simulink model "V2X_Core_SRI_coding_rate_symbol"  (R2023b)
settings: Solver=ode23tb  StartTime=0.0  StopTime=50  MaxStep=1e-2  RelTol=1e-3  AbsTol=1e-3
StopFcn:
  | run('saving.m')
values from neighbouring files (symbols this model uses):
  b = 1.6    [a2024_v2x_matlab_6veh.m]
  m = 2000    [a2024_v2x_matlab_6veh.m]
  mEgo = 1500    [a2024_v2x_matlab_6veh.m]
  Mode = 1    [a2024_v2x_matlab_6veh.m]    (also in v2x_matlab.m; v2x_matlabV2.m; v2x_matlab_6veh.m; v2x_matlab_R.m)
  RefSpeed = 90/3.6    (= 25)    [v2x_matlabV2.m]    (also in v2x_matlab_R.m)
  RelDistThreshold = 300    [v2x_matlabV2.m]    (also in v2x_matlab_R.m)
  s = RandStream("dsfmt19937","Seed",15)    [v2x_matlab.m]
  sampleTime = 0.1    [a2024_v2x_matlab_6veh.m]    (also in v2x_matlab.m; v2x_matlabV2.m; v2x_matlab_6veh.m; v2x_matlab_R.m)
  waypoints = [egoWP(:,2) egoWP(:,1), zeroforwp]    [a2024_v2x_matlab_6veh.m]    (also in misc.m = data.data.ActorSpecifications(1,1).Waypoints(:,[1,2]); v2x_matlab.m = data.data.ActorSpecifications(1,1).Waypoints(:,[1,2]); v2x_matlabV2.m = [5 -1.6 0; v2x_matlab_R.m = [5 -1.6 0)
  ZeroActors = struct(     'ActorID',0,     'Position', [1000 1000 1000],      'Velocity', [0 0 0],      'Roll', 0,      'Pitch', 0,      'Yaw', 0,      'AngularVelocity', [0 0 0])    [v2x_matlabV2.m]    (also in v2x_matlab_R.m)
undefined symbols (not defined in the file or in its folder): Battery, Brakes, Control, DiscIntNeverNeededParam, doppler, Drivetrain, ElectricMotor, Env, FB_flag, Init, SNR_value_list, Vehicle, Wheels
libraries: simulink x45, commofdm x29, commdigbbndam3 x15, commchan3 x14, simulink_extras x13, commcnvcod2 x12, commdigbbndpm3 x11, commblkintrlv2 x10, dspmathops x6, sharedtransform x6, autolibutils x6, autolibsharedcoupling x4
(part 5 of 8)

== system V2X_Core_SRI_coding_rate_symbol/DSRC/Subsystem/2//3 64 QAM ==
  Bits : Inport
  Pilot : Inport  Port=2
  Constant2 : Constant  Value=[zeros(24,1)']  SampleTime=-1
  Convolutional Encoder1 : commcnvcod2/Convolutional Encoder  trellis=poly2trellis(7, [171 133])  opMode=Truncated (reset every frame)  DelayedResetAction=on  hasIniStPort=off  hasFinStPort=off  usePuncVector=on  punctureVector=[1; 1; 0; 1]  reset=Unused parameter value
      settings: LibrarySourceBlock=|
      | commhdlcnvcod/Convolutional
      | Encoder
  Gain : Gain  Gain=1/sqrt(5)
  OFDM Modulator1 : commofdm/OFDM Modulator  StatePerturbationForJacobian=1.0e-05  FFTLength=64  NumGuardBandCarriers=[6; 5]  InsertDCNull=on  PilotInputPort=on  PilotCarrierIndices=[12; 26; 40; 54]  CyclicPrefixLength=16  Windowing=off  WindowLength=1  OversamplingFactor=1  NumSymbols=2  NumTransmitAntennas=1  SimulateUsing=Interpreted execution
  Random Interleaver : commblkintrlv2/Random Interleaver  StatePerturbationForJacobian=1.0e-05  N=432  seed=12345
  Rectangular QAM Modulator Baseband2 : commdigbbndam3/Rectangular QAM Modulator Baseband  M=2^6  InType=Bit  Enc=Gray  Mapping=[0:15]  PowType=Average Power  MinDist=2  AvgPow=1  PeakPow=42  Ph=0  outDtype=double  outWordLen=16  outUDDataType=sfix(16)  outFracLenMode=Best precision  outFracLen=15  outDataTypeStr=double  outLastDataTypeStr=double
      settings: LibrarySourceBlock=|
      | commhdldigbbndam/Rectangular QAM
      | Modulator
      | Baseband
  Reshape : Reshape  OutputDimensionality=Customize  OutputDimensions=[48,2]
  Vector Concatenate : Concatenate
  Modulated : Outport
  wires:
  Convolutional Encoder1/1 -> Random Interleaver/1
  OFDM Modulator1/1 -> Modulated/1  "OFDM modulated"
  Pilot/1 -> OFDM Modulator1/2
  Vector Concatenate/1 -> Reshape/1  "After QAM Mod"
  Constant2/1 -> Vector Concatenate/2
  Random Interleaver/1 -> Rectangular QAM Modulator Baseband2/1
  Reshape/1 -> OFDM Modulator1/1
  Bits/1 -> Convolutional Encoder1/1
  Rectangular QAM Modulator Baseband2/1 -> Gain/1
  Gain/1 -> Vector Concatenate/1

== system V2X_Core_SRI_coding_rate_symbol/DSRC/Subsystem/2//3 64 QAM1 ==
  Bits : Inport
  Pilot : Inport  Port=2
  Constant2 : Constant  Value=[zeros(24,1)']  SampleTime=-1
  Convolutional Encoder1 : commcnvcod2/Convolutional Encoder  trellis=poly2trellis(7, [171 133])  opMode=Truncated (reset every frame)  DelayedResetAction=on  hasIniStPort=off  hasFinStPort=off  usePuncVector=on  punctureVector=[1; 1; 0; 1]  reset=Unused parameter value
      settings: LibrarySourceBlock=|
      | commhdlcnvcod/Convolutional
      | Encoder
  OFDM Modulator1 : commofdm/OFDM Modulator  StatePerturbationForJacobian=1.0e-05  FFTLength=64  NumGuardBandCarriers=[6; 5]  InsertDCNull=on  PilotInputPort=on  PilotCarrierIndices=[12; 26; 40; 54]  CyclicPrefixLength=16  Windowing=off  WindowLength=1  OversamplingFactor=1  NumSymbols=2  NumTransmitAntennas=1  SimulateUsing=Interpreted execution
  OFDM Modulator2 : commofdm/OFDM Modulator  Commented=on  StatePerturbationForJacobian=1.0e-05  FFTLength=1024  NumGuardBandCarriers=[0;0]  InsertDCNull=on  PilotInputPort=on  PilotCarrierIndices=[128; 256; 384; 640; 768; 896]  CyclicPrefixLength=256  Windowing=off  WindowLength=16  OversamplingFactor=3  NumSymbols=1  NumTransmitAntennas=1  SimulateUsing=Interpreted execution
  Rectangular QAM Modulator Baseband2 : commdigbbndam3/Rectangular QAM Modulator Baseband  M=2^6  InType=Bit  Enc=Gray  Mapping=[0:15]  PowType=Average Power  MinDist=2  AvgPow=42  PeakPow=1  Ph=0  outDtype=double  outWordLen=16  outUDDataType=sfix(16)  outFracLenMode=Best precision  outFracLen=15  outDataTypeStr=double  outLastDataTypeStr=double
      settings: LibrarySourceBlock=|
      | commhdldigbbndam/Rectangular QAM
      | Modulator
      | Baseband
  Reshape : Reshape  OutputDimensionality=Customize  OutputDimensions=[48,2]
  Vector Concatenate : Concatenate
  Modulated : Outport
  wires:
  Constant2/1 -> Vector Concatenate/2
  Vector Concatenate/1 -> Reshape/1  "After QAM Mod"
  Pilot/1 -> OFDM Modulator1/2
  Rectangular QAM Modulator Baseband2/1 -> Vector Concatenate/1
  OFDM Modulator1/1 -> Modulated/1  "OFDM modulated"
  Bits/1 -> Convolutional Encoder1/1
  Convolutional Encoder1/1 -> Rectangular QAM Modulator Baseband2/1
  Reshape/1 -> OFDM Modulator1/1

== system V2X_Core_SRI_coding_rate_symbol/DSRC/Subsystem/3//4 64 QAM ==
  Bits : Inport
  Pilot : Inport  Port=2
  Constant2 : Constant  Value=[zeros(32,1)']  SampleTime=-1
  Convolutional Encoder1 : commcnvcod2/Convolutional Encoder  trellis=poly2trellis(7, [171 133])  opMode=Truncated (reset every frame)  DelayedResetAction=on  hasIniStPort=off  hasFinStPort=off  usePuncVector=on  punctureVector=[1; 1; 0; 1; 1; 0]  reset=Unused parameter value
      settings: LibrarySourceBlock=|
      | commhdlcnvcod/Convolutional
      | Encoder
  OFDM Modulator1 : commofdm/OFDM Modulator  StatePerturbationForJacobian=1.0e-05  FFTLength=64  NumGuardBandCarriers=[6; 5]  InsertDCNull=on  PilotInputPort=on  PilotCarrierIndices=[12; 26; 40; 54]  CyclicPrefixLength=16  Windowing=off  WindowLength=1  OversamplingFactor=1  NumSymbols=2  NumTransmitAntennas=1  SimulateUsing=Interpreted execution
  Random Interleaver : commblkintrlv2/Random Interleaver  StatePerturbationForJacobian=1.0e-05  N=384  seed=12345
  Rectangular QAM Modulator Baseband2 : commdigbbndam3/Rectangular QAM Modulator Baseband  M=2^6  InType=Bit  Enc=Gray  Mapping=[0:15]  PowType=Average Power  MinDist=2  AvgPow=0.2  PeakPow=1  Ph=0  outDtype=double  outWordLen=16  outUDDataType=sfix(16)  outFracLenMode=Best precision  outFracLen=15  outDataTypeStr=double  outLastDataTypeStr=double
      settings: LibrarySourceBlock=|
      | commhdldigbbndam/Rectangular QAM
      | Modulator
      | Baseband
  Reshape : Reshape  OutputDimensionality=Customize  OutputDimensions=[48,2]
  Vector Concatenate : Concatenate
  Modulated : Outport
  wires:
  Constant2/1 -> Vector Concatenate/2
  Vector Concatenate/1 -> Reshape/1  "After QAM Mod"
  Pilot/1 -> OFDM Modulator1/2
  Rectangular QAM Modulator Baseband2/1 -> Vector Concatenate/1
  OFDM Modulator1/1 -> Modulated/1  "OFDM modulated"
  Bits/1 -> Convolutional Encoder1/1
  Convolutional Encoder1/1 -> Random Interleaver/1
  Random Interleaver/1 -> Rectangular QAM Modulator Baseband2/1
  Reshape/1 -> OFDM Modulator1/1

== system V2X_Core_SRI_coding_rate_symbol/DSRC/Subsystem/3//4 QPSK ==
  Bits : Inport
  Pilot : Inport  Port=2
  Constant : Constant  Commented=on  Value=zeros(0,1)
  Convolutional Encoder1 : commcnvcod2/Convolutional Encoder  trellis=poly2trellis(7, [171 133])  opMode=Truncated (reset every frame)  DelayedResetAction=on  hasIniStPort=off  hasFinStPort=off  usePuncVector=on  punctureVector=[1; 1; 0; 1; 1; 0]  reset=Unused parameter value
      settings: LibrarySourceBlock=|
      | commhdlcnvcod/Convolutional
      | Encoder
  Gain : Gain  Gain=1/sqrt(5)
  OFDM Modulator : commofdm/OFDM Modulator  StatePerturbationForJacobian=1.0e-05  FFTLength=64  NumGuardBandCarriers=[6; 5]  InsertDCNull=on  PilotInputPort=on  PilotCarrierIndices=[12; 26; 40; 54]  CyclicPrefixLength=16  Windowing=off  WindowLength=1  OversamplingFactor=1  NumSymbols=4  NumTransmitAntennas=1  SimulateUsing=Interpreted execution
  QPSK Modulator Baseband : commdigbbndpm3/QPSK Modulator Baseband  InType=Bit  Enc=Gray  Ph=pi/4  outDtype=double  outWordLen=16  outUDDataType=sfix(16)  outFracLenMode=Best precision  outFracLen=15  outDataTypeStr=double  outLastDataTypeStr=double
      settings: LibrarySourceBlock=|
      | commhdldigbbndpm/QPSK
      | Modulator
      | Baseband
  Random Interleaver : commblkintrlv2/Random Interleaver  StatePerturbationForJacobian=1.0e-05  N=384  seed=12345
  Reshape : Reshape  OutputDimensionality=Customize  OutputDimensions=[48,4]
  Vector Concatenate : Concatenate  Commented=on
  Modulated : Outport
  wires:
  OFDM Modulator/1 -> Modulated/1  "OFDM modulated"
  Pilot/1 -> OFDM Modulator/2
  Bits/1 -> Convolutional Encoder1/1
  Constant/1 -> Vector Concatenate/2
  Convolutional Encoder1/1 -> Random Interleaver/1
  Random Interleaver/1 -> QPSK Modulator Baseband/1
  QPSK Modulator Baseband/1 -> Gain/1
  Reshape/1 -> OFDM Modulator/1
  Gain/1 -> Reshape/1

== system V2X_Core_SRI_coding_rate_symbol/DSRC/Subsystem3/1//2 QPSK ==
  Output : Inport
  Bit to Integer Converter2 : simulink/Logic and Bit Operations/Bit to Integer Converter  nbits=16  bitOrder=MSB first  signedOutputValues=Signed  outDtype=int16  outDtypeSigned=int16
  Display : Display
  OFDM Demodulator1 : commofdm/OFDM Demodulator  StatePerturbationForJacobian=1.0e-05  FFTLength=64  NumGuardBandCarriers=[6; 5]  RemoveDCCarrier=on  PilotOutputPort=on  PilotCarrierIndices=[12; 26; 40; 54]  CyclicPrefixLength=16  OversamplingFactor=1  NumSymbols=6  NumReceiveAntennas=1  SimulateUsing=Interpreted execution
  QPSK Demodulator Baseband : commdigbbndpm3/QPSK Demodulator Baseband  OutType=Bit  DecType=Hard decision  VarSource=Dialog  Variance=1  Dec=Gray  Ph=pi/4  outDtype1=Inherit via internal rule  outDtype2=Inherit via internal rule  derotateFactorWordLen=16  derotateFactorDataTypeStr=Inherit: Same word length as input  derotateFactorLastDataTypeStr=Inherit: Same word length as input
      settings: LibrarySourceBlock=|
      | commhdldigbbndpm/QPSK
      | Demodulator
      | Baseband
  Random Deinterleaver : commblkintrlv2/Random Deinterleaver  StatePerturbationForJacobian=1.0e-05  N=576  seed=12345
  Reshape : Reshape
  Selector : Selector  InputPortWidth=288  IndexOptions=Index vector (dialog)  Indices=[1:288]  OutputSizes=1
  Viterbi Decoder : commcnvcod2/Viterbi Decoder  trellis=poly2trellis(7, [171 133])  isPunctured=off  punctureVector=[1; 1; 0; 1; 1; 0]  erasures=off  dectype=Hard decision  nsdecb=4  runSigValErrCheck=off  tbdepth=30  opmode=Truncated  reset=off  delayedResetAction=on  smWordLength=16  outDataType=Smallest unsigned integer
      settings: LibrarySourceBlock=commhdlcnvcod/Viterbi Decoder
  Modulated : Outport
  wires:
  OFDM Demodulator1/2 -> Display/1
  OFDM Demodulator1/1 -> Reshape/1  "Before QAM Demod"
  Output/1 -> OFDM Demodulator1/1
  QPSK Demodulator Baseband/1 -> Random Deinterleaver/1
  Selector/1 -> QPSK Demodulator Baseband/1
  Bit to Integer Converter2/1 -> Modulated/1
  Viterbi Decoder/1 -> Bit to Integer Converter2/1
  Random Deinterleaver/1 -> Viterbi Decoder/1
  Reshape/1 -> Selector/1

== system V2X_Core_SRI_coding_rate_symbol/DSRC/Subsystem3/1//2 QPSK1 ==
  Output : Inport
  Bit to Integer Converter2 : simulink/Logic and Bit Operations/Bit to Integer Converter  nbits=16  bitOrder=MSB first  signedOutputValues=Signed  outDtype=int16  outDtypeSigned=int16
  Display : Display
  OFDM Demodulator1 : commofdm/OFDM Demodulator  Commented=on  StatePerturbationForJacobian=1.0e-05  FFTLength=64  NumGuardBandCarriers=[0; 0]  RemoveDCCarrier=on  PilotOutputPort=on  PilotCarrierIndices=[12; 26; 40; 54]  CyclicPrefixLength=32  OversamplingFactor=3  NumSymbols=1  NumReceiveAntennas=1  SimulateUsing=Interpreted execution
  OFDM Demodulator2 : commofdm/OFDM Demodulator  StatePerturbationForJacobian=1.0e-05  FFTLength=64  NumGuardBandCarriers=[6; 5]  RemoveDCCarrier=on  PilotOutputPort=on  PilotCarrierIndices=[12; 26; 40; 54]  CyclicPrefixLength=16  OversamplingFactor=1  NumSymbols=6  NumReceiveAntennas=1  SimulateUsing=Interpreted execution
  QPSK Demodulator Baseband : commdigbbndpm3/QPSK Demodulator Baseband  OutType=Bit  DecType=Hard decision  VarSource=Dialog  Variance=1  Dec=Gray  Ph=pi/4  outDtype1=Inherit via internal rule  outDtype2=Inherit via internal rule  derotateFactorWordLen=16  derotateFactorDataTypeStr=Inherit: Same word length as input  derotateFactorLastDataTypeStr=Inherit: Same word length as input
      settings: LibrarySourceBlock=|
      | commhdldigbbndpm/QPSK
      | Demodulator
      | Baseband
  Random Deinterleaver : commblkintrlv2/Random Deinterleaver  StatePerturbationForJacobian=1.0e-05  N=576  seed=12345
  Reshape : Reshape
  Selector : Selector  InputPortWidth=288  IndexOptions=Index vector (dialog)  Indices=[1:288]  OutputSizes=1
  Viterbi Decoder : commcnvcod2/Viterbi Decoder  trellis=poly2trellis(7, [171 133])  isPunctured=off  punctureVector=[1; 1; 0; 1; 1; 0]  erasures=off  dectype=Hard decision  nsdecb=4  runSigValErrCheck=off  tbdepth=30  opmode=Truncated  reset=off  delayedResetAction=on  smWordLength=16  outDataType=Smallest unsigned integer
      settings: LibrarySourceBlock=commhdlcnvcod/Viterbi Decoder
  Modulated : Outport
  wires:
  Viterbi Decoder/1 -> Bit to Integer Converter2/1
  Bit to Integer Converter2/1 -> Modulated/1
  Selector/1 -> QPSK Demodulator Baseband/1
  QPSK Demodulator Baseband/1 -> Random Deinterleaver/1
  Output/1 -> OFDM Demodulator2/1
  OFDM Demodulator2/1 -> Reshape/1  "Before QAM Demod"
  OFDM Demodulator2/2 -> Display/1
  Reshape/1 -> Selector/1
  Random Deinterleaver/1 -> Viterbi Decoder/1

== system V2X_Core_SRI_coding_rate_symbol/DSRC/Subsystem3/2//3 64 QAM ==
  Output : Inport
  Bit to Integer Converter2 : simulink/Logic and Bit Operations/Bit to Integer Converter  nbits=16  bitOrder=MSB first  signedOutputValues=Signed  outDtype=int16  outDtypeSigned=int16
  Display : Display
  Display1 : Display
  MATLAB Function3 : MATLAB Function  Commented=on  TreatAsAtomicUnit=on
  OFDM Demodulator1 : commofdm/OFDM Demodulator  StatePerturbationForJacobian=1.0e-05  FFTLength=64  NumGuardBandCarriers=[6; 5]  RemoveDCCarrier=on  PilotOutputPort=on  PilotCarrierIndices=[12; 26; 40; 54]  CyclicPrefixLength=16  OversamplingFactor=1  NumSymbols=2  NumReceiveAntennas=1  SimulateUsing=Interpreted execution
  Random Deinterleaver : commblkintrlv2/Random Deinterleaver  StatePerturbationForJacobian=1.0e-05  N=432  seed=12345
  Rectangular QAM Demodulator Baseband2 : commdigbbndam3/Rectangular QAM Demodulator Baseband  M=2^6  OutType=Bit  DecType=Hard decision  VarSource=Dialog  Variance=1  Dec=Gray  Mapping=[0:15]  PowType=Average Power  MinDist=2  AvgPow=0.2  PeakPow=1  Ph=0  outDtype1=int16  outDtype2=int16  derotateFactorWordLen=16  derotateFactorDataTypeStr=Inherit: Same word length as input  derotateFactorLastDataTypeStr=Inherit: Same word length as input  denormFactorWordLen=16  denormFactorDataTypeStr=Inherit: Same word length as input  denormFactorLastDataTypeStr=Inherit: Same word length as input  prodOutWordLen=32  prodOutOverflowMode=Wrap  prodOutRoundingMode=Floor  prodOutOvFlMode=off  prodOutOvFlModeLastStrValue=off  sumWordLen=32
      settings: LibrarySourceBlock=|
      | commhdldigbbndam/Rectangular QAM
      | Demodulator
      | Baseband
  Reshape : Reshape
  Selector : Selector  InputPortWidth=96  IndexOptions=Index vector (dialog)  Indices=[1:72]  OutputSizes=1
  Viterbi Decoder : commcnvcod2/Viterbi Decoder  trellis=poly2trellis(7, [171 133])  isPunctured=on  punctureVector=[1; 1; 0; 1]  erasures=off  dectype=Hard decision  nsdecb=4  runSigValErrCheck=off  tbdepth=30  opmode=Truncated  reset=off  delayedResetAction=on  smWordLength=16  outDataType=Smallest unsigned integer
      settings: LibrarySourceBlock=commhdlcnvcod/Viterbi Decoder
  Modulated : Outport
  wires:
  Rectangular QAM Demodulator Baseband2/1 -> Random Deinterleaver/1
  Bit to Integer Converter2/1 -> Modulated/1, Display1/1
  OFDM Demodulator1/1 -> Reshape/1  "Before QAM Demod"
  Selector/1 -> Rectangular QAM Demodulator Baseband2/1
  Output/1 -> OFDM Demodulator1/1
  OFDM Demodulator1/2 -> Display/1
  Random Deinterleaver/1 -> Viterbi Decoder/1
  Reshape/1 -> Selector/1
  Viterbi Decoder/1 -> Bit to Integer Converter2/1

== system V2X_Core_SRI_coding_rate_symbol/DSRC/Subsystem3/2//3 64 QAM1 ==
  Output : Inport
  Bit to Integer Converter2 : simulink/Logic and Bit Operations/Bit to Integer Converter  nbits=16  bitOrder=MSB first  signedOutputValues=Signed  outDtype=int16  outDtypeSigned=int16
  Display : Display
  Display1 : Display
  MATLAB Function3 : MATLAB Function  Commented=on  TreatAsAtomicUnit=on
  OFDM Demodulator : commofdm/OFDM Demodulator  StatePerturbationForJacobian=1.0e-05  FFTLength=64  NumGuardBandCarriers=[6; 5]  RemoveDCCarrier=on  PilotOutputPort=on  PilotCarrierIndices=[12; 26; 40; 54]  CyclicPrefixLength=16  OversamplingFactor=1  NumSymbols=2  NumReceiveAntennas=1  SimulateUsing=Interpreted execution
  OFDM Demodulator1 : commofdm/OFDM Demodulator  Commented=on  StatePerturbationForJacobian=1.0e-05  FFTLength=1024  NumGuardBandCarriers=[0; 0]  RemoveDCCarrier=on  PilotOutputPort=on  PilotCarrierIndices=[128; 256; 384; 640; 768; 896]  CyclicPrefixLength=256  OversamplingFactor=3  NumSymbols=1  NumReceiveAntennas=1  SimulateUsing=Interpreted execution
  Rectangular QAM Demodulator Baseband2 : commdigbbndam3/Rectangular QAM Demodulator Baseband  M=2^6  OutType=Bit  DecType=Hard decision  VarSource=Dialog  Variance=1  Dec=Gray  Mapping=[0:15]  PowType=Average Power  MinDist=2  AvgPow=42  PeakPow=1  Ph=0  outDtype1=int16  outDtype2=int16  derotateFactorWordLen=16  derotateFactorDataTypeStr=Inherit: Same word length as input  derotateFactorLastDataTypeStr=Inherit: Same word length as input  denormFactorWordLen=16  denormFactorDataTypeStr=Inherit: Same word length as input  denormFactorLastDataTypeStr=Inherit: Same word length as input  prodOutWordLen=32  prodOutOverflowMode=Wrap  prodOutRoundingMode=Floor  prodOutOvFlMode=off  prodOutOvFlModeLastStrValue=off  sumWordLen=32
      settings: LibrarySourceBlock=|
      | commhdldigbbndam/Rectangular QAM
      | Demodulator
      | Baseband
  Reshape : Reshape
  Selector : Selector  InputPortWidth=96  IndexOptions=Index vector (dialog)  Indices=[1:72]  OutputSizes=1
  Viterbi Decoder : commcnvcod2/Viterbi Decoder  trellis=poly2trellis(7, [171 133])  isPunctured=on  punctureVector=[1; 1; 0; 1]  erasures=off  dectype=Hard decision  nsdecb=4  runSigValErrCheck=off  tbdepth=30  opmode=Truncated  reset=off  delayedResetAction=on  smWordLength=16  outDataType=Smallest unsigned integer
      settings: LibrarySourceBlock=commhdlcnvcod/Viterbi Decoder
  Modulated : Outport
  wires:
  OFDM Demodulator/2 -> Display/1
  Output/1 -> OFDM Demodulator/1
  Selector/1 -> Rectangular QAM Demodulator Baseband2/1
  Bit to Integer Converter2/1 -> Display1/1, Modulated/1
  Rectangular QAM Demodulator Baseband2/1 -> Viterbi Decoder/1
  Viterbi Decoder/1 -> Bit to Integer Converter2/1
  OFDM Demodulator/1 -> Reshape/1  "Before QAM Demod"
  Reshape/1 -> Selector/1

== system V2X_Core_SRI_coding_rate_symbol/DSRC/Subsystem3/3//4 64 QAM ==
  Output : Inport
  Bit to Integer Converter2 : simulink/Logic and Bit Operations/Bit to Integer Converter  nbits=16  bitOrder=MSB first  signedOutputValues=Signed  outDtype=int16  outDtypeSigned=int16
  Display : Display
  Display1 : Display
  MATLAB Function3 : MATLAB Function  Commented=on  TreatAsAtomicUnit=on
  OFDM Demodulator1 : commofdm/OFDM Demodulator  StatePerturbationForJacobian=1.0e-05  FFTLength=64  NumGuardBandCarriers=[6; 5]  RemoveDCCarrier=on  PilotOutputPort=on  PilotCarrierIndices=[12; 26; 40; 54]  CyclicPrefixLength=16  OversamplingFactor=1  NumSymbols=2  NumReceiveAntennas=1  SimulateUsing=Interpreted execution
  Random Deinterleaver : commblkintrlv2/Random Deinterleaver  StatePerturbationForJacobian=1.0e-05  N=384  seed=12345
  Rectangular QAM Demodulator Baseband2 : commdigbbndam3/Rectangular QAM Demodulator Baseband  M=2^6  OutType=Bit  DecType=Hard decision  VarSource=Dialog  Variance=1  Dec=Gray  Mapping=[0:15]  PowType=Average Power  MinDist=2  AvgPow=0.2  PeakPow=1  Ph=0  outDtype1=int16  outDtype2=int16  derotateFactorWordLen=16  derotateFactorDataTypeStr=Inherit: Same word length as input  derotateFactorLastDataTypeStr=Inherit: Same word length as input  denormFactorWordLen=16  denormFactorDataTypeStr=Inherit: Same word length as input  denormFactorLastDataTypeStr=Inherit: Same word length as input  prodOutWordLen=32  prodOutOverflowMode=Wrap  prodOutRoundingMode=Floor  prodOutOvFlMode=off  prodOutOvFlModeLastStrValue=off  sumWordLen=32
      settings: LibrarySourceBlock=|
      | commhdldigbbndam/Rectangular QAM
      | Demodulator
      | Baseband
  Reshape : Reshape
  Selector : Selector  InputPortWidth=96  IndexOptions=Index vector (dialog)  Indices=[1:64]  OutputSizes=1
  Viterbi Decoder : commcnvcod2/Viterbi Decoder  trellis=poly2trellis(7, [171 133])  isPunctured=on  punctureVector=[1; 1; 0; 1; 1; 0]  erasures=off  dectype=Hard decision  nsdecb=4  runSigValErrCheck=off  tbdepth=60  opmode=Truncated  reset=off  delayedResetAction=on  smWordLength=16  outDataType=Smallest unsigned integer
      settings: LibrarySourceBlock=commhdlcnvcod/Viterbi Decoder
  Modulated : Outport
  wires:
  OFDM Demodulator1/2 -> Display/1
  Output/1 -> OFDM Demodulator1/1
  Selector/1 -> Rectangular QAM Demodulator Baseband2/1
  OFDM Demodulator1/1 -> Reshape/1  "Before QAM Demod"
  Bit to Integer Converter2/1 -> Display1/1, Modulated/1
  Rectangular QAM Demodulator Baseband2/1 -> Random Deinterleaver/1
  Viterbi Decoder/1 -> Bit to Integer Converter2/1
  Random Deinterleaver/1 -> Viterbi Decoder/1
  Reshape/1 -> Selector/1

== system V2X_Core_SRI_coding_rate_symbol/DSRC/Subsystem3/3//4 QPSK ==
  Output : Inport
  Bit to Integer Converter2 : simulink/Logic and Bit Operations/Bit to Integer Converter  nbits=16  bitOrder=MSB first  signedOutputValues=Signed  outDtype=int16  outDtypeSigned=int16
  Display : Display
  OFDM Demodulator1 : commofdm/OFDM Demodulator  StatePerturbationForJacobian=1.0e-05  FFTLength=64  NumGuardBandCarriers=[6; 5]  RemoveDCCarrier=on  PilotOutputPort=on  PilotCarrierIndices=[12; 26; 40; 54]  CyclicPrefixLength=16  OversamplingFactor=1  NumSymbols=4  NumReceiveAntennas=1  SimulateUsing=Interpreted execution
  QPSK Demodulator Baseband : commdigbbndpm3/QPSK Demodulator Baseband  OutType=Bit  DecType=Hard decision  VarSource=Dialog  Variance=1  Dec=Gray  Ph=pi/4  outDtype1=Inherit via internal rule  outDtype2=Inherit via internal rule  derotateFactorWordLen=16  derotateFactorDataTypeStr=Inherit: Same word length as input  derotateFactorLastDataTypeStr=Inherit: Same word length as input
      settings: LibrarySourceBlock=|
      | commhdldigbbndpm/QPSK
      | Demodulator
      | Baseband
  Random Deinterleaver : commblkintrlv2/Random Deinterleaver  StatePerturbationForJacobian=1.0e-05  N=384  seed=12345
  Reshape : Reshape
  Selector : Selector  InputPortWidth=192  IndexOptions=Index vector (dialog)  Indices=[1:192]  OutputSizes=1
  Viterbi Decoder : commcnvcod2/Viterbi Decoder  trellis=poly2trellis(7, [171 133])  isPunctured=on  punctureVector=[1; 1; 0; 1; 1; 0]  erasures=off  dectype=Hard decision  nsdecb=4  runSigValErrCheck=off  tbdepth=60  opmode=Truncated  reset=off  delayedResetAction=on  smWordLength=16  outDataType=Smallest unsigned integer
      settings: LibrarySourceBlock=commhdlcnvcod/Viterbi Decoder
  Modulated : Outport
  wires:
  Viterbi Decoder/1 -> Bit to Integer Converter2/1
  Bit to Integer Converter2/1 -> Modulated/1
  Selector/1 -> QPSK Demodulator Baseband/1
  QPSK Demodulator Baseband/1 -> Random Deinterleaver/1
  Output/1 -> OFDM Demodulator1/1
  OFDM Demodulator1/1 -> Reshape/1  "Before QAM Demod"
  OFDM Demodulator1/2 -> Display/1
  Random Deinterleaver/1 -> Viterbi Decoder/1
  Reshape/1 -> Selector/1

== system V2X_Core_SRI_coding_rate_symbol/DSRC/Subsystem3/If Action Subsystem ==
  In1 : Inport
  Action Port : ActionPort  ActionPortLabel=case [ 1 ]:
  Out1 : Outport
  wires:
  In1/1 -> Out1/1

== system V2X_Core_SRI_coding_rate_symbol/DSRC/Subsystem3/If Action Subsystem1 ==
  In1 : Inport
  Action Port : ActionPort  ActionPortLabel=case [ 2 ]:
  Out1 : Outport
  wires:
  In1/1 -> Out1/1

== system V2X_Core_SRI_coding_rate_symbol/DSRC/Subsystem3/If Action Subsystem2 ==
  Actors : Inport
  Action Port : ActionPort  ActionPortLabel=case [ 3 ]:
  Out1 : Outport
  wires:
  Actors/1 -> Out1/1

== system V2X_Core_SRI_coding_rate_symbol/DSRC/Subsystem3/If Action Subsystem3 ==
  Actors : Inport
  Action Port : ActionPort  ActionPortLabel=case [ 4 ]:
  Out1 : Outport
  wires:
  Actors/1 -> Out1/1

== system V2X_Core_SRI_coding_rate_symbol/DSRC/Subsystem3/If Action Subsystem4 ==
  Actors : Inport
  Action Port : ActionPort  ActionPortLabel=case [ 5 ]:
  Out1 : Outport
  wires:
  Actors/1 -> Out1/1

== system V2X_Core_SRI_coding_rate_symbol/DSRC/Subsystem3/If Action Subsystem5 ==
  Actors : Inport
  Action Port : ActionPort  ActionPortLabel=case [ 6 ]:
  Out1 : Outport
  wires:
  Actors/1 -> Out1/1

== system V2X_Core_SRI_coding_rate_symbol/DSRC/Subsystem4/1//2 QPSK ==
  Bits : Inport
  Pilot : Inport  Port=2
  Constant : Constant  Value=zeros(3,1)
  Gain : Gain  Gain=1/2
  OFDM Modulator1 : commofdm/OFDM Modulator  StatePerturbationForJacobian=1.0e-05  FFTLength=128  NumGuardBandCarriers=[0;0]  InsertDCNull=on  PilotInputPort=on  PilotCarrierIndices=[24; 52; 80; 108]  CyclicPrefixLength=32  Windowing=off  WindowLength=16  OversamplingFactor=3  NumSymbols=1  NumTransmitAntennas=1  SimulateUsing=Interpreted execution
  QPSK Modulator Baseband : commdigbbndpm3/QPSK Modulator Baseband  InType=Bit  Enc=Gray  Ph=pi/4  outDtype=double  outWordLen=16  outUDDataType=sfix(16)  outFracLenMode=Best precision  outFracLen=15  outDataTypeStr=double  outLastDataTypeStr=double
      settings: LibrarySourceBlock=|
      | commhdldigbbndpm/QPSK
      | Modulator
      | Baseband
  Vector Concatenate : Concatenate
  Modulated : Outport
  wires:
  Constant/1 -> Vector Concatenate/2
  Vector Concatenate/1 -> OFDM Modulator1/1
  QPSK Modulator Baseband/1 -> Gain/1
  Bits/1 -> QPSK Modulator Baseband/1
  Gain/1 -> Vector Concatenate/1
  Pilot/1 -> OFDM Modulator1/2
  OFDM Modulator1/1 -> Modulated/1  "OFDM modulated"

== system V2X_Core_SRI_coding_rate_symbol/DSRC/Subsystem4/64 QAM ==
  Bits : Inport
  Pilot : Inport  Port=2
  Constant2 : Constant  Value=[zeros(19,1)']  SampleTime=-1
  OFDM Modulator : commofdm/OFDM Modulator  StatePerturbationForJacobian=1.0e-05  FFTLength=64  NumGuardBandCarriers=[0;0]  InsertDCNull=on  PilotInputPort=on  PilotCarrierIndices=[12; 26; 40; 54]  CyclicPrefixLength=32  Windowing=off  WindowLength=16  OversamplingFactor=3  NumSymbols=1  NumTransmitAntennas=1  SimulateUsing=Interpreted execution
  Rectangular QAM Modulator Baseband2 : commdigbbndam3/Rectangular QAM Modulator Baseband  M=2^6  InType=Bit  Enc=Gray  Mapping=[0:15]  PowType=Average Power  MinDist=2  AvgPow=P_Signal  PeakPow=1  Ph=0  outDtype=double  outWordLen=16  outUDDataType=sfix(16)  outFracLenMode=Best precision  outFracLen=15  outDataTypeStr=double  outLastDataTypeStr=double
      settings: LibrarySourceBlock=|
      | commhdldigbbndam/Rectangular QAM
      | Modulator
      | Baseband
  Vector Concatenate : Concatenate
  Modulated : Outport
  wires:
  OFDM Modulator/1 -> Modulated/1  "OFDM modulated"
  Bits/1 -> Rectangular QAM Modulator Baseband2/1
  Rectangular QAM Modulator Baseband2/1 -> Vector Concatenate/1
  Pilot/1 -> OFDM Modulator/2
  Vector Concatenate/1 -> OFDM Modulator/1  "After QAM Mod"
  Constant2/1 -> Vector Concatenate/2

== system V2X_Core_SRI_coding_rate_symbol/DSRC/Subsystem5/1//2 QPSK ==
  Bits : Inport
  Pilot : Inport  Port=2
  Constant : Constant  Value=zeros(3,1)
  Gain : Gain  Gain=1/2
  OFDM Modulator1 : commofdm/OFDM Modulator  StatePerturbationForJacobian=1.0e-05  FFTLength=128  NumGuardBandCarriers=[0;0]  InsertDCNull=on  PilotInputPort=on  PilotCarrierIndices=[24; 52; 80; 108]  CyclicPrefixLength=32  Windowing=off  WindowLength=16  OversamplingFactor=3  NumSymbols=1  NumTransmitAntennas=1  SimulateUsing=Interpreted execution
  QPSK Modulator Baseband : commdigbbndpm3/QPSK Modulator Baseband  InType=Bit  Enc=Gray  Ph=pi/4  outDtype=double  outWordLen=16  outUDDataType=sfix(16)  outFracLenMode=Best precision  outFracLen=15  outDataTypeStr=double  outLastDataTypeStr=double
      settings: LibrarySourceBlock=|
      | commhdldigbbndpm/QPSK
      | Modulator
      | Baseband
  Vector Concatenate : Concatenate
  Modulated : Outport
  wires:
  OFDM Modulator1/1 -> Modulated/1  "OFDM modulated"
  Pilot/1 -> OFDM Modulator1/2
  Gain/1 -> Vector Concatenate/1
  Bits/1 -> QPSK Modulator Baseband/1
  QPSK Modulator Baseband/1 -> Gain/1
  Vector Concatenate/1 -> OFDM Modulator1/1
  Constant/1 -> Vector Concatenate/2

== system V2X_Core_SRI_coding_rate_symbol/DSRC/Subsystem5/64 QAM ==
  Bits : Inport
  Pilot : Inport  Port=2
  Constant2 : Constant  Value=[zeros(19,1)']  SampleTime=-1
  OFDM Modulator : commofdm/OFDM Modulator  StatePerturbationForJacobian=1.0e-05  FFTLength=64  NumGuardBandCarriers=[0;0]  InsertDCNull=on  PilotInputPort=on  PilotCarrierIndices=[12; 26; 40; 54]  CyclicPrefixLength=32  Windowing=off  WindowLength=16  OversamplingFactor=3  NumSymbols=1  NumTransmitAntennas=1  SimulateUsing=Interpreted execution
  Rectangular QAM Modulator Baseband2 : commdigbbndam3/Rectangular QAM Modulator Baseband  M=2^6  InType=Bit  Enc=Gray  Mapping=[0:15]  PowType=Average Power  MinDist=2  AvgPow=P_Signal  PeakPow=1  Ph=0  outDtype=double  outWordLen=16  outUDDataType=sfix(16)  outFracLenMode=Best precision  outFracLen=15  outDataTypeStr=double  outLastDataTypeStr=double
      settings: LibrarySourceBlock=|
      | commhdldigbbndam/Rectangular QAM
      | Modulator
      | Baseband
  Vector Concatenate : Concatenate
  Modulated : Outport
  wires:
  Constant2/1 -> Vector Concatenate/2
  Vector Concatenate/1 -> OFDM Modulator/1  "After QAM Mod"
  Pilot/1 -> OFDM Modulator/2
  Rectangular QAM Modulator Baseband2/1 -> Vector Concatenate/1
  Bits/1 -> Rectangular QAM Modulator Baseband2/1
  OFDM Modulator/1 -> Modulated/1  "OFDM modulated"

== system V2X_Core_SRI_coding_rate_symbol/DSRC/Subsystem6/1//2 QPSK ==
  Bits : Inport
  Pilot : Inport  Port=2
  Constant : Constant  Value=zeros(3,1)
  Gain : Gain  Gain=1/2
  OFDM Modulator1 : commofdm/OFDM Modulator  StatePerturbationForJacobian=1.0e-05  FFTLength=128  NumGuardBandCarriers=[0;0]  InsertDCNull=on  PilotInputPort=on  PilotCarrierIndices=[24; 52; 80; 108]  CyclicPrefixLength=32  Windowing=off  WindowLength=16  OversamplingFactor=3  NumSymbols=1  NumTransmitAntennas=1  SimulateUsing=Interpreted execution
  QPSK Modulator Baseband : commdigbbndpm3/QPSK Modulator Baseband  InType=Bit  Enc=Gray  Ph=pi/4  outDtype=double  outWordLen=16  outUDDataType=sfix(16)  outFracLenMode=Best precision  outFracLen=15  outDataTypeStr=double  outLastDataTypeStr=double
      settings: LibrarySourceBlock=|
      | commhdldigbbndpm/QPSK
      | Modulator
      | Baseband
  Vector Concatenate : Concatenate
  Modulated : Outport
  wires:
  Constant/1 -> Vector Concatenate/2
  Vector Concatenate/1 -> OFDM Modulator1/1
  QPSK Modulator Baseband/1 -> Gain/1
  Bits/1 -> QPSK Modulator Baseband/1
  Gain/1 -> Vector Concatenate/1
  Pilot/1 -> OFDM Modulator1/2
  OFDM Modulator1/1 -> Modulated/1  "OFDM modulated"

== system V2X_Core_SRI_coding_rate_symbol/DSRC/Subsystem6/64 QAM ==
  Bits : Inport
  Pilot : Inport  Port=2
  Constant2 : Constant  Value=[zeros(19,1)']  SampleTime=-1
  OFDM Modulator : commofdm/OFDM Modulator  StatePerturbationForJacobian=1.0e-05  FFTLength=64  NumGuardBandCarriers=[0;0]  InsertDCNull=on  PilotInputPort=on  PilotCarrierIndices=[12; 26; 40; 54]  CyclicPrefixLength=32  Windowing=off  WindowLength=16  OversamplingFactor=3  NumSymbols=1  NumTransmitAntennas=1  SimulateUsing=Interpreted execution
  Rectangular QAM Modulator Baseband2 : commdigbbndam3/Rectangular QAM Modulator Baseband  M=2^6  InType=Bit  Enc=Gray  Mapping=[0:15]  PowType=Average Power  MinDist=2  AvgPow=P_Signal  PeakPow=1  Ph=0  outDtype=double  outWordLen=16  outUDDataType=sfix(16)  outFracLenMode=Best precision  outFracLen=15  outDataTypeStr=double  outLastDataTypeStr=double
      settings: LibrarySourceBlock=|
      | commhdldigbbndam/Rectangular QAM
      | Modulator
      | Baseband
  Vector Concatenate : Concatenate
  Modulated : Outport
  wires:
  OFDM Modulator/1 -> Modulated/1  "OFDM modulated"
  Bits/1 -> Rectangular QAM Modulator Baseband2/1
  Rectangular QAM Modulator Baseband2/1 -> Vector Concatenate/1
  Pilot/1 -> OFDM Modulator/2
  Vector Concatenate/1 -> OFDM Modulator/1  "After QAM Mod"
  Constant2/1 -> Vector Concatenate/2

== system V2X_Core_SRI_coding_rate_symbol/DSRC/Subsystem7/1//2 QPSK ==
  Bits : Inport
  Pilot : Inport  Port=2
  Constant : Constant  Value=zeros(3,1)
  Gain : Gain  Gain=1/2
  OFDM Modulator1 : commofdm/OFDM Modulator  StatePerturbationForJacobian=1.0e-05  FFTLength=128  NumGuardBandCarriers=[0;0]  InsertDCNull=on  PilotInputPort=on  PilotCarrierIndices=[24; 52; 80; 108]  CyclicPrefixLength=32  Windowing=off  WindowLength=16  OversamplingFactor=3  NumSymbols=1  NumTransmitAntennas=1  SimulateUsing=Interpreted execution
  QPSK Modulator Baseband : commdigbbndpm3/QPSK Modulator Baseband  InType=Bit  Enc=Gray  Ph=pi/4  outDtype=double  outWordLen=16  outUDDataType=sfix(16)  outFracLenMode=Best precision  outFracLen=15  outDataTypeStr=double  outLastDataTypeStr=double
      settings: LibrarySourceBlock=|
      | commhdldigbbndpm/QPSK
      | Modulator
      | Baseband
  Vector Concatenate : Concatenate
  Modulated : Outport
  wires:
  OFDM Modulator1/1 -> Modulated/1  "OFDM modulated"
  Pilot/1 -> OFDM Modulator1/2
  Gain/1 -> Vector Concatenate/1
  Bits/1 -> QPSK Modulator Baseband/1
  QPSK Modulator Baseband/1 -> Gain/1
  Vector Concatenate/1 -> OFDM Modulator1/1
  Constant/1 -> Vector Concatenate/2

== system V2X_Core_SRI_coding_rate_symbol/DSRC/Subsystem7/64 QAM ==
  Bits : Inport
  Pilot : Inport  Port=2
  Constant2 : Constant  Value=[zeros(19,1)']  SampleTime=-1
  OFDM Modulator : commofdm/OFDM Modulator  StatePerturbationForJacobian=1.0e-05  FFTLength=64  NumGuardBandCarriers=[0;0]  InsertDCNull=on  PilotInputPort=on  PilotCarrierIndices=[12; 26; 40; 54]  CyclicPrefixLength=32  Windowing=off  WindowLength=16  OversamplingFactor=3  NumSymbols=1  NumTransmitAntennas=1  SimulateUsing=Interpreted execution
  Rectangular QAM Modulator Baseband2 : commdigbbndam3/Rectangular QAM Modulator Baseband  M=2^6  InType=Bit  Enc=Gray  Mapping=[0:15]  PowType=Average Power  MinDist=2  AvgPow=P_Signal  PeakPow=1  Ph=0  outDtype=double  outWordLen=16  outUDDataType=sfix(16)  outFracLenMode=Best precision  outFracLen=15  outDataTypeStr=double  outLastDataTypeStr=double
      settings: LibrarySourceBlock=|
      | commhdldigbbndam/Rectangular QAM
      | Modulator
      | Baseband
  Vector Concatenate : Concatenate
  Modulated : Outport
  wires:
  Constant2/1 -> Vector Concatenate/2
  Vector Concatenate/1 -> OFDM Modulator/1  "After QAM Mod"
  Pilot/1 -> OFDM Modulator/2
  Rectangular QAM Modulator Baseband2/1 -> Vector Concatenate/1
  Bits/1 -> Rectangular QAM Modulator Baseband2/1
  OFDM Modulator/1 -> Modulated/1  "OFDM modulated"

== system V2X_Core_SRI_coding_rate_symbol/DSRC/Subsystem8/1//2 QPSK ==
  Bits : Inport
  Pilot : Inport  Port=2
  Constant : Constant  Value=zeros(3,1)
  Gain : Gain  Gain=1/2
  OFDM Modulator1 : commofdm/OFDM Modulator  StatePerturbationForJacobian=1.0e-05  FFTLength=128  NumGuardBandCarriers=[0;0]  InsertDCNull=on  PilotInputPort=on  PilotCarrierIndices=[24; 52; 80; 108]  CyclicPrefixLength=32  Windowing=off  WindowLength=16  OversamplingFactor=3  NumSymbols=1  NumTransmitAntennas=1  SimulateUsing=Interpreted execution
  QPSK Modulator Baseband : commdigbbndpm3/QPSK Modulator Baseband  InType=Bit  Enc=Gray  Ph=pi/4  outDtype=double  outWordLen=16  outUDDataType=sfix(16)  outFracLenMode=Best precision  outFracLen=15  outDataTypeStr=double  outLastDataTypeStr=double
      settings: LibrarySourceBlock=|
      | commhdldigbbndpm/QPSK
      | Modulator
      | Baseband
  Vector Concatenate : Concatenate
  Modulated : Outport
  wires:
  Constant/1 -> Vector Concatenate/2
  Vector Concatenate/1 -> OFDM Modulator1/1
  QPSK Modulator Baseband/1 -> Gain/1
  Bits/1 -> QPSK Modulator Baseband/1
  Gain/1 -> Vector Concatenate/1
  Pilot/1 -> OFDM Modulator1/2
  OFDM Modulator1/1 -> Modulated/1  "OFDM modulated"

== system V2X_Core_SRI_coding_rate_symbol/DSRC/Subsystem8/64 QAM ==
  Bits : Inport
  Pilot : Inport  Port=2
  Constant2 : Constant  Value=[zeros(19,1)']  SampleTime=-1
  OFDM Modulator : commofdm/OFDM Modulator  StatePerturbationForJacobian=1.0e-05  FFTLength=64  NumGuardBandCarriers=[0;0]  InsertDCNull=on  PilotInputPort=on  PilotCarrierIndices=[12; 26; 40; 54]  CyclicPrefixLength=32  Windowing=off  WindowLength=16  OversamplingFactor=3  NumSymbols=1  NumTransmitAntennas=1  SimulateUsing=Interpreted execution
  Rectangular QAM Modulator Baseband2 : commdigbbndam3/Rectangular QAM Modulator Baseband  M=2^6  InType=Bit  Enc=Gray  Mapping=[0:15]  PowType=Average Power  MinDist=2  AvgPow=P_Signal  PeakPow=1  Ph=0  outDtype=double  outWordLen=16  outUDDataType=sfix(16)  outFracLenMode=Best precision  outFracLen=15  outDataTypeStr=double  outLastDataTypeStr=double
      settings: LibrarySourceBlock=|
      | commhdldigbbndam/Rectangular QAM
      | Modulator
      | Baseband
  Vector Concatenate : Concatenate
  Modulated : Outport
  wires:
  OFDM Modulator/1 -> Modulated/1  "OFDM modulated"
  Bits/1 -> Rectangular QAM Modulator Baseband2/1
  Rectangular QAM Modulator Baseband2/1 -> Vector Concatenate/1
  Pilot/1 -> OFDM Modulator/2
  Vector Concatenate/1 -> OFDM Modulator/1  "After QAM Mod"
  Constant2/1 -> Vector Concatenate/2

== system V2X_Core_SRI_coding_rate_symbol/VehicleDynamic/AccelerationToTrq/CalculateIntendedTorque ==
  IntendedLongAcc[m/s**2] : Inport
  UnloadedTireRadius[m] : Inport  Port=2
  OverallMass[kg] : Inport  Port=3
  EngInrt[kg*m**2] : Inport  Port=4
  WheelRotAxisInrt[kg*m**2] : Inport  Port=5
  TireMaxRollResistanceTrq[Nm] : Inport  Port=6
  AeroFrc(VehSys)[N] : Inport  Port=7
  TorqueRatio[-] : Inport  Port=8
  MinEngTrq[Nm] : Inport  Port=9
  Acceleration Resistance Torque : Subsystem
  Driving Resistance Torque : Subsystem
  Reference Torque : Subsystem
  IntendedTrq[Nm] : Outport  VectorParamsAs1DForOutWhenUnconnected=off
  wires:
  Acceleration Resistance Torque/1(AccResistanceTrq[Nm]) -> Reference Torque/1(AccResistanceTrq[Nm])
  TireMaxRollResistanceTrq[Nm]/1 -> Driving Resistance Torque/2(TireMaxRollResistanceTrq[Nm])
  WheelRotAxisInrt[kg*m**2]/1 -> Acceleration Resistance Torque/3(WheelRotAxisInrt[kg*m**2])
  MinEngTrq[Nm]/1 -> Reference Torque/4(MinEngTrq[Nm])
  IntendedLongAcc[m/s**2]/1 -> Acceleration Resistance Torque/1(IntendedLongAcc[m/s**2])
  AeroFrc(VehSys)[N]/1 -> Driving Resistance Torque/3(AeroFrc(VehSys)[N])
  OverallMass[kg]/1 -> Acceleration Resistance Torque/4(OverallMass[kg])
  UnloadedTireRadius[m]/1 -> Driving Resistance Torque/1(UnloadedTireRadius[m]), Acceleration Resistance Torque/5(UnloadedTireRadius[m])
  EngInrt[kg*m**2]/1 -> Acceleration Resistance Torque/2(EngInrt[kg*m**2])
  Reference Torque/1(IntendedTrq[Nm]) -> IntendedTrq[Nm]/1
  TorqueRatio[-]/1 -> Reference Torque/2(TorqueRatio[-]), Acceleration Resistance Torque/6(TorqueRatio[-])
  Driving Resistance Torque/1(DrivingResistanceTrq[Nm]) -> Reference Torque/3(DrivingResistanceTrq[Nm])

== system V2X_Core_SRI_coding_rate_symbol/VehicleDynamic/AccelerationToTrq/CalculateMainBrakePressure ==
  IntendedBrakeTrq[Nm] : Inport
  StandstillSwitch[0;1] : Inport  Port=2
  LongVehSpd[m/s] : Inport  Port=3
  MaxMainBrakePress[Pa] : Inport  Port=4
  BrakeTrqPressRatio[m**3] : Inport  Port=5
  Constant : Constant  Commented=on  Value=0
  Constant1 : Constant  Value=0
  Divide : Product  Inputs=*/
  Divide1 : Product  Commented=on  Inputs=**
  Lookup Table : Lookup  Commented=on  InputValues=[-500 0.3 10 500]/3.6  Table=[0.7 0.7 0 0]  SaturateOnIntegerOverflow=off
  NonZero : Subsystem
  Rate Limiter : RateLimiter  Commented=on  RisingSlewLimit=0.02  FallingSlewLimit=-0.05  SampleTimeMode=inherited
  Saturation Dynamic : simulink/Discontinuities/Saturation Dynamic  OutMin=[]  OutMax=[]  OutDataTypeStr=Inherit: Same as second input  OutDataType=fixdt(1, 16)  OutScaling=2^-10  DoSatur=off
  Subtract : Sum
  Sum of Elements1 : Sum  Inputs=+
  Switch1 : Switch  Commented=on  Criteria=u2 > Threshold  SaturateOnIntegerOverflow=off  InputSameDT=off
  IntendedMainBrakePress[Pa] : Outport  VectorParamsAs1DForOutWhenUnconnected=off
  wires:
  Saturation Dynamic/1 -> IntendedMainBrakePress[Pa]/1
  Switch1/1 -> Rate Limiter/1
  NonZero/1(Output) -> Divide/2
  IntendedBrakeTrq[Nm]/1 -> Divide/1
  MaxMainBrakePress[Pa]/1 -> Divide1/2, Saturation Dynamic/1
  Lookup Table/1 -> Switch1/1
  Rate Limiter/1 -> Divide1/1
  Divide/1 -> Subtract/1
  Sum of Elements1/1 -> NonZero/1(Input)
  LongVehSpd[m/s]/1 -> Lookup Table/1
  Constant1/1 -> Saturation Dynamic/3
  Constant/1 -> Switch1/3
  Divide1/1 -> Subtract/2  "AdditionalMainBrakePress for standstill"
  StandstillSwitch[0;1]/1 -> Switch1/2
  Subtract/1 -> Saturation Dynamic/2
  BrakeTrqPressRatio[m**3]/1 -> Sum of Elements1/1

== system V2X_Core_SRI_coding_rate_symbol/VehicleDynamic/AccelerationToTrq/TorqueSplitter ==
  "IntendedTrq[Nm] " : Inport
  ZeroAccPedalTrq[Nm] : Inport  Port=2
  TorqueRatio[-] : Inport  Port=3
  FullAccPedalTrq[Nm] : Inport  Port=4
  Add : Sum  Inputs=+-
  Gain : Gain  Gain=-1
  MinMax1 : MinMax  Inputs=2
  Product : Product  RndMeth=Zero
  Saturation Dynamic : simulink/Discontinuities/Saturation Dynamic  OutMin=[]  OutMax=[]  OutDataTypeStr=Inherit: Same as second input  OutDataType=fixdt(1, 16)  OutScaling=2^-10  DoSatur=off
  IntendedDriveTrq[Nm] : Outport  VectorParamsAs1DForOutWhenUnconnected=off
  IntendedBrakeTrq[Nm] : Outport  Port=2  VectorParamsAs1DForOutWhenUnconnected=off
  wires:
  Saturation Dynamic/1 -> IntendedDriveTrq[Nm]/1
  Product/1 -> Gain/1
  FullAccPedalTrq[Nm]/1 -> Saturation Dynamic/1
  ZeroAccPedalTrq[Nm]/1 -> Add/2, MinMax1/2, Saturation Dynamic/3
  TorqueRatio[-]/1 -> Product/2
  "IntendedTrq[Nm] "/1 -> MinMax1/1, Saturation Dynamic/2
  Gain/1 -> IntendedBrakeTrq[Nm]/1
  Add/1 -> Product/1
  MinMax1/1 -> Add/1

== system V2X_Core_SRI_coding_rate_symbol/VehicleDynamic/DrivetrainControlUnit/Accel Pedal to Traction Wheel Torque Request ==
  note: Convert Accelerator Pedal Position to Torque Command
      | using Motor Torque Speed Curve
  AccelPdl : Inport
  EMSpd : Inport  Port=2
  MaxEMTrqVsSpd : Lookup_n-D  NumberOfTableDimensions=1  BreakpointsForDimension1=ElectricMotor.SpeedVector*30/pi  Table=ElectricMotor.TorqueVector  ExtrapMethod=Clip  UseLastTableValue=on  InternalRulePriority=Speed  OutDataTypeStr=Inherit: Inherit from 'Table data'  RndMeth=Simplest
  Product1 : Product
  rads_to_rpm : Gain  Gain=30/pi
  TrqCmd : Outport  VectorParamsAs1DForOutWhenUnconnected=off
  wires:
  Product1/1 -> TrqCmd/1
  MaxEMTrqVsSpd/1 -> Product1/2
  AccelPdl/1 -> Product1/1
  EMSpd/1 -> rads_to_rpm/1
  rads_to_rpm/1 -> MaxEMTrqVsSpd/1

== system V2X_Core_SRI_coding_rate_symbol/VehicleDynamic/DrivetrainControlUnit/Brake Pedal to Total Braking Pressure Request ==
  BcuBrkPrsCmd : Inport
  Park : Inport  Port=2
  Front Bias : Constant  Value=Brakes.BiasFront
  Gain4 : Gain  Gain=Brakes.MaxPressure
  Mux : Mux
  Product : Product
  Rear Bias : Constant  Value=Brakes.BiasRear
  Terminator : Terminator
  BrkPrsReq : Outport  VectorParamsAs1DForOutWhenUnconnected=off
  wires:
  BcuBrkPrsCmd/1 -> Product/2
  Mux/1 -> Product/1
  Rear Bias/1 -> Mux/4, Mux/3
  Front Bias/1 -> Mux/1, Mux/2
  Gain4/1 -> BrkPrsReq/1
  Product/1 -> Gain4/1
  Park/1 -> Terminator/1

== system V2X_Core_SRI_coding_rate_symbol/VehicleDynamic/DrivetrainControlUnit/Motor Torque Arbitration and Power Management ==
  EMTrqCmdTrac : Inport
  AccelPdl : Inport  Port=2
  BattPwrDisChrgLmt : Inport  Port=3
  "BattPwrChrgLmt " : Inport  Port=4
  EMSpd : Inport  Port=5
  SOC : Inport  Port=6
  EMTrqCmdRegen : Inport  Port=7
  Accel Decel Switch : Switch  Criteria=u2 > Threshold  SaturateOnIntegerOverflow=off  InputSameDT=off
  Compare To Constant : simulink/Logic and Bit Operations/Compare To Constant  relop=>  const=0  OutDataTypeStr=boolean
  Power Management : Subsystem
  EMTrqCmdFinal : Outport  VectorParamsAs1DForOutWhenUnconnected=off
  wires:
  AccelPdl/1 -> Compare To Constant/1
  EMTrqCmdRegen/1 -> Accel Decel Switch/3
  EMTrqCmdTrac/1 -> Accel Decel Switch/1
  Power Management/1(EMTrqCmdFinal) -> EMTrqCmdFinal/1
  Accel Decel Switch/1 -> Power Management/4(EMTrqCmd)
  BattPwrDisChrgLmt/1 -> Power Management/1(BattPwrDischrgLmt)
  "BattPwrChrgLmt "/1 -> Power Management/2(BattPwrChrgLmt)
  EMSpd/1 -> Power Management/3(EMSpd)
  Compare To Constant/1 -> Accel Decel Switch/2
  SOC/1 -> Power Management/5(SOC)

== system V2X_Core_SRI_coding_rate_symbol/VehicleDynamic/DrivetrainControlUnit/Power Limit Calculations ==
  note: Use Current Limits from BMS to calculate
      | discharge and charge power limits
  PackVolt : Inport
  BMSDischrgCurrLmt : Inport  Port=2
  BMSChrgCurrLmt : Inport  Port=3
  Data Type Conversion : DataTypeConversion  SaturateOnIntegerOverflow=off  RndMeth=Floor
  Data Type Conversion1 : DataTypeConversion  SaturateOnIntegerOverflow=off  RndMeth=Floor
  Gain : Gain  Gain=-1
  Gain1 : Gain  Gain=-1
  Product : Product
  Product1 : Product
  BattPwrDischrgLmt : Outport  VectorParamsAs1DForOutWhenUnconnected=off
  BattPwrChrgLmt : Outport  Port=2  VectorParamsAs1DForOutWhenUnconnected=off
  wires:
  Gain/1 -> Product1/2
  Gain1/1 -> Product/2
  Product/1 -> Data Type Conversion1/1
  Product1/1 -> Data Type Conversion/1
  PackVolt/1 -> Product/1, Product1/1
  BMSChrgCurrLmt/1 -> Gain/1
  BMSDischrgCurrLmt/1 -> Gain1/1
  Data Type Conversion/1 -> BattPwrChrgLmt/1
  Data Type Conversion1/1 -> BattPwrDischrgLmt/1
